simulink model "model_disturbance"  (R2019a)
settings: Solver=ode14x  StartTime=0.0  StopTime=10  FixedStep=0.01  RelTol=1e-3
undefined symbols (not defined in the file or in its folder): iokd, ioki, iokp, k, Kd, Kp, Lambda, tau
settings Model: Creator=Bo Shang  LastModifiedBy=standard
settings DataIOCC: LimitDataPoints=on  SaveFormat=Array  SaveState=on  ReturnWorkspaceOutputs=off
settings OptimizationCC: BlockReduction=off  BooleanDataType=off  LifeSpan=inf
settings DebuggingCC: SaveWithParameterizedLinksMsg=none  UnderspecifiedInitializationDetection=Classic  MergeDetectMultiDrivingBlocksExec=none  SignalResolutionControl=TryResolveAllWithWarning  PregeneratedLibrarySubsystemCodeDiagnostic=none  SFUnexpectedBacktrackingDiag=warning  SFNoUnconditionalDefaultTransitionDiag=warning  SFExecutionAtInitializationDiag=none  ArithmeticOperatorsInVariantConditions=warning
settings HardwareCC: ProdBitPerPointer=32  ProdBitPerSizeT=32  ProdBitPerPtrDiffT=32  ProdLargestAtomicFloat=None  ProdIntDivRoundTo=Undefined  ProdEndianess=Unspecified  ProdWordSize=32  ProdHWDeviceType=32-bit Generic  TargetUnknown=on
settings ModelReferenceCC: PropagateSignalLabelsOutOfModel=off
settings SFSimCC: SimUseLocalCustomCode=off
settings RTWCC: RTWUseLocalCustomCode=off
settings CodeAppCC: StateflowObjectComments=on
settings GRTTargetCC: TargetLangStandard=C89/C90 (ANSI)  GeneratePreprocessorConditionals=Disable all
settings ConfigComp: CovMetricSettings=dw  CovHtmlReporting=on  CovSaveCumulativeToWorkspaceVar=on  CovSaveSingleToWorkspaceVar=on  CovExternalEMLEnable=off  CovSFcnEnable=off

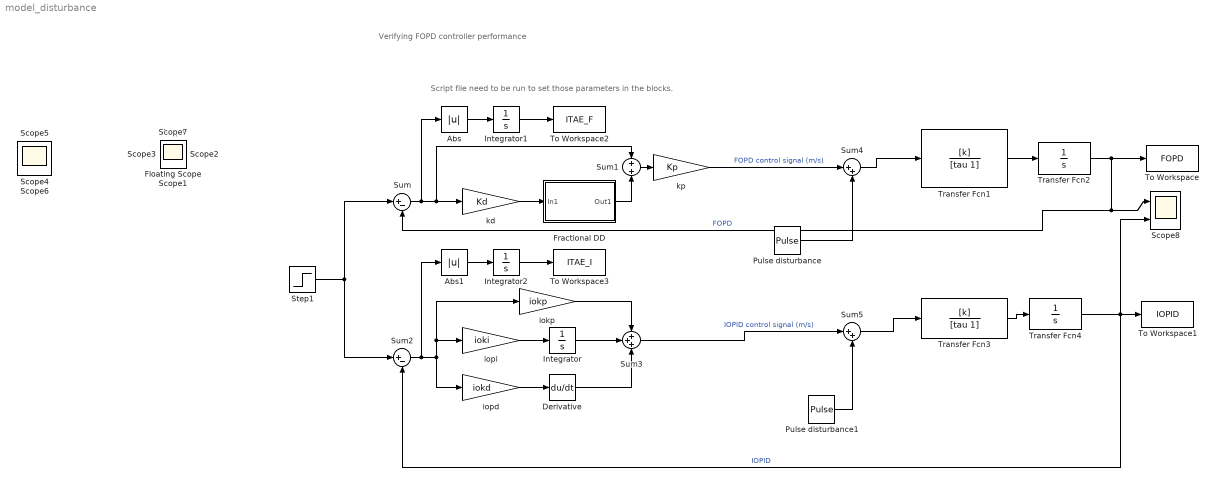
== system model_disturbance ==
  note: Verifying FOPD controller performance
  note: Script file need to be run to set those parameters in the blocks.
  Abs : Abs
  Abs1 : Abs
  Derivative : Derivative  CoefficientInTFapproximation=0
  Fractional DD : Subsystem  mask{gam=Lambda, ww=[0.001,1000], n=4}
      mask prompts: gam "Derivative order gamma"; ww "Frequency range [wb,wh]"; n "Apprixmation order"
      mask init:
      | wb=ww(1); wh=ww(2); G=zz(gam,n,wb,wh);
      | num=G.num{1}; den=G.den{1}; T=1/wh; str='Fractional\n';
      | if isnumeric(gam)
      | 	if gam>0, str=[str, 'Der  s^' num2str(gam) ];
      | 	else, str=[str, 'Int  s^{' num2str(gam) '}']; end
      | else, str=[str, 'Der  s^gam']; end
      mask Display: disp(str)
  Integrator : Integrator
  Integrator1 : Integrator
  Integrator2 : Integrator
  Pulse disturbance : DiscretePulseGenerator  PulseType=Time based  Amplitude=0.1  Period=20  PulseWidth=4  PhaseDelay=1
  Pulse disturbance1 : DiscretePulseGenerator  PulseType=Time based  Amplitude=0.1  Period=20  PulseWidth=4  PhaseDelay=1
  Scope8 : Scope  NumInputPorts=2
  Step1 : Step  Time=0  After=0  SampleTime=0
  Sum : Sum  Inputs=|+-
  Sum1 : Sum  Inputs=+|+
  Sum2 : Sum  Inputs=|+-
  Sum3 : Sum  Inputs=+++
  Sum4 : Sum  Inputs=|++
  Sum5 : Sum  Inputs=|++
  To Workspace : ToWorkspace  VariableName=FOPD  SaveFormat=Timeseries  SampleTime=-1
  To Workspace1 : ToWorkspace  VariableName=IOPID  SaveFormat=Timeseries  SampleTime=-1
  To Workspace2 : ToWorkspace  VariableName=ITAE_F  SaveFormat=Timeseries  SampleTime=-1
  To Workspace3 : ToWorkspace  VariableName=ITAE_I  SaveFormat=Timeseries  SampleTime=-1
  Transfer Fcn1 : TransferFcn  Numerator=[k]  Denominator=[tau 1]
  Transfer Fcn2 : TransferFcn  Denominator=[1 0]
  Transfer Fcn3 : TransferFcn  Numerator=[k]  Denominator=[tau 1]
  Transfer Fcn4 : TransferFcn  Denominator=[1 0]
  iokp : Gain  Gain=iokp
  iopd : Gain  Gain=iokd
  iopi : Gain  Gain=ioki
  kd : Gain  Gain=Kd
  kp : Gain  Gain=Kp
  Floating Scope : Scope
  Scope{,1..7} (8 alike) : Scope
  wires:
  Fractional DD/1(Out1) -> Sum1/2
  kd/1 -> Fractional DD/1(In1)
  Sum1/1 -> kp/1
  Sum/1 -> Abs/1, Sum1/1, kd/1
  Transfer Fcn1/1 -> Transfer Fcn2/1
  Transfer Fcn2/1 -> To Workspace/1, Scope8/1, Sum/2  "FOPD"
  Transfer Fcn3/1 -> Transfer Fcn4/1
  Transfer Fcn4/1 -> To Workspace1/1, Scope8/2, Sum2/2  "IOPID"
  Step1/1 -> Sum/1, Sum2/1
  Derivative/1 -> Sum3/3
  iopd/1 -> Derivative/1
  Sum3/1 -> Sum5/1  "IOPID control signal (m/s)"
  iokp/1 -> Sum3/1
  iopi/1 -> Integrator/1
  Integrator/1 -> Sum3/2
  Integrator1/1 -> To Workspace2/1
  Abs/1 -> Integrator1/1
  Sum2/1 -> Abs1/1, iokp/1, iopi/1, iopd/1
  Integrator2/1 -> To Workspace3/1
  Abs1/1 -> Integrator2/1
  Pulse disturbance/1 -> Sum4/2
  Sum4/1 -> Transfer Fcn1/1
  kp/1 -> Sum4/1  "FOPD control signal (m/s)"
  Pulse disturbance1/1 -> Sum5/2
  Sum5/1 -> Transfer Fcn3/1

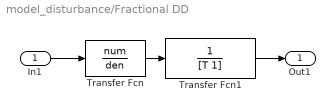
== system model_disturbance/Fractional DD ==
  In1 : Inport
  Transfer Fcn : TransferFcn  Numerator=num  Denominator=den
  Transfer Fcn1 : TransferFcn  Numerator=1  Denominator=[T 1]
  Out1 : Outport
  wires:
  Transfer Fcn1/1 -> Out1/1
  Transfer Fcn/1 -> Transfer Fcn1/1
  In1/1 -> Transfer Fcn/1
